simulink model "slGTC_3gdl"  (Simulink 9.0)
settings: Solver=ode45  StartTime=0.0  StopTime=1.5  MaxStep=1e-3  RelTol=1e-8  EnableMultiTasking=on
values from neighbouring files (symbols this model uses):
  Duracion = 0.5    [test.m]
  N_puntos = 50    [test.m]
  Tini = 0.5    [test.m]
  XYZfin = CinematicaDirecta([0.5 0.5 0.5])    [test.m]
  XYZini = CinematicaDirecta([0 0 0])    [test.m]
settings Model: Creator=Manuel G. Ortega  LastModifiedBy=Raúl  ExtModeTrigMode=oneshot  ExtModeArmWhenConnect=off
settings DataIOCC: SignalLoggingSaveFormat=ModelDataLogs
settings OptimizationCC: BooleanDataType=off  ExpressionDepthLimit=2147483647  InitFltsAndDblsToZero=on
settings DebuggingCC: SaveWithParameterizedLinksMsg=none  SignalResolutionControl=TryResolveAllWithWarning  MultiTaskDSMMsg=warning  MultiTaskCondExecSysMsg=none  FcnCallInpInsideContextMsg=warning  StateNameClashWarn=warning  StrictBusMsg=None
settings HardwareCC: TargetUnknown=on
settings GRTTargetCC: TargetFcnLib=ansi_tfl_tmw.mat  GeneratePreprocessorConditionals=Disable all  CombineOutputUpdateFcns=off  GRTInterface=on
settings ConfigComp: CovSFcnEnable=off

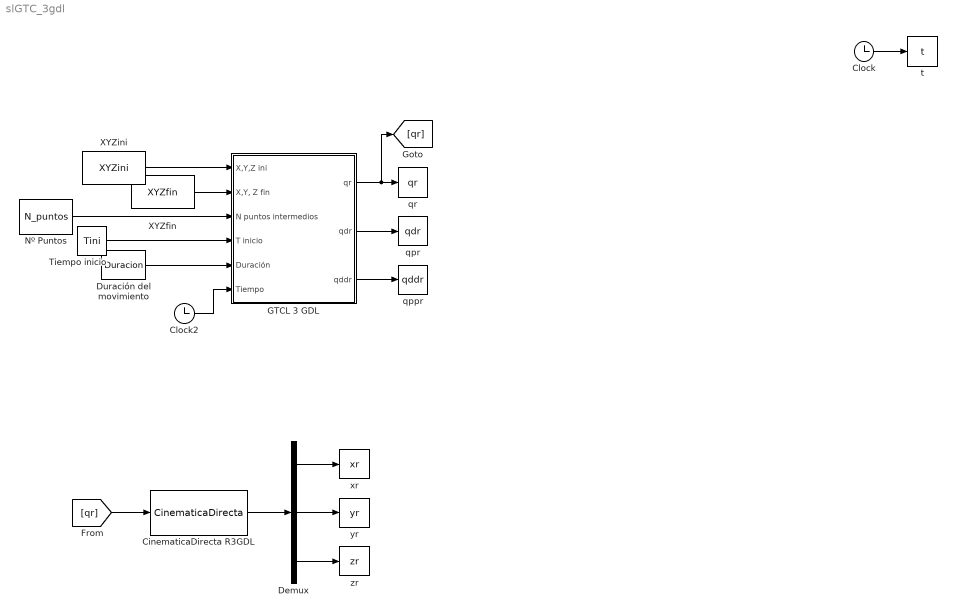
== system slGTC_3gdl ==
  CinematicaDirecta R3GDL : MATLABFcn  MATLABFcn=CinematicaDirecta
  Clock : Clock
  Clock2 : Clock
  Demux : Demux  Outputs=3
  Duración del movimiento : Constant  Value=Duracion
  GTCL 3 GDL : Subsystem
  Nº Puntos : Constant  Value=N_puntos
  Tiempo inicio : Constant  Value=Tini
  XYZfin : Constant  Value=XYZfin
  XYZini : Constant  Value=XYZini
  qppr : ToWorkspace  VariableName=qddr  SampleTime=-1
  qpr : ToWorkspace  VariableName=qdr  SampleTime=-1
  qr : ToWorkspace  VariableName=qr  SampleTime=-1
  t : ToWorkspace  VariableName=t  SampleTime=-1
  xr : ToWorkspace  VariableName=xr  SampleTime=-1
  yr : ToWorkspace  VariableName=yr  SampleTime=-1
  zr : ToWorkspace  VariableName=zr  SampleTime=-1
  wires:
  Clock/1 -> t/1
  Duración del movimiento/1 -> GTCL 3 GDL/5(Duración)
  [qr] -> CinematicaDirecta R3GDL/1
  CinematicaDirecta R3GDL/1 -> Demux/1
  Demux/1 -> xr/1
  Demux/2 -> yr/1
  Demux/3 -> zr/1
  GTCL 3 GDL/2(qdr) -> qpr/1
  GTCL 3 GDL/1(qr) -> [qr], qr/1
  GTCL 3 GDL/3(qddr) -> qppr/1
  Clock2/1 -> GTCL 3 GDL/6(Tiempo)
  Nº Puntos/1 -> GTCL 3 GDL/3(N puntos intermedios)
  Tiempo inicio/1 -> GTCL 3 GDL/4(T inicio)
  XYZfin/1 -> GTCL 3 GDL/2("X,Y, Z fin")
  XYZini/1 -> GTCL 3 GDL/1(X,Y,Z ini)

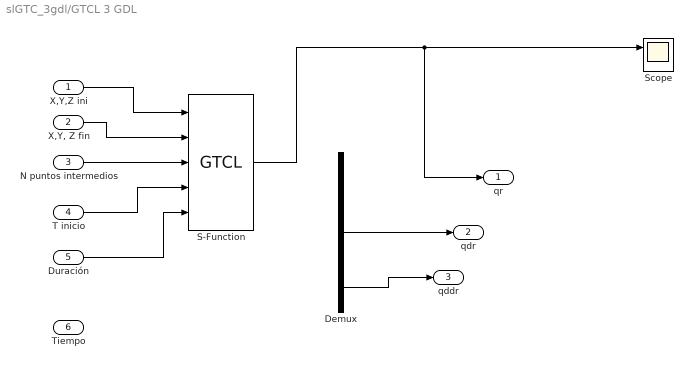
== system slGTC_3gdl/GTCL 3 GDL ==
  X,Y,Z ini : Inport
  "X,Y, Z fin" : Inport  Port=2
  N puntos intermedios : Inport  Port=3
  T inicio : Inport  Port=4
  Duración : Inport  Port=5
  Tiempo : Inport  Port=6
  Demux : Demux  Outputs=3
  S-Function : S-Function  FunctionName=GTCL  SFunctionDeploymentMode=off  EnableBusSupport=off
  Scope : Scope  NumInputPorts=2
  qr : Outport
  qdr : Outport  Port=2
  qddr : Outport  Port=3
  wires:
  Demux/2 -> qdr/1
  Demux/3 -> qddr/1
  S-Function/1 -> qr/1, Scope/1
  X,Y,Z ini/1 -> S-Function/1
  "X,Y, Z fin"/1 -> S-Function/2
  N puntos intermedios/1 -> S-Function/3
  T inicio/1 -> S-Function/4
  Duración/1 -> S-Function/5
